simulink model "supercaps_dcbus_control"  (Simulink 7.2)
settings: Solver=ode45  StartTime=0.0  StopTime=1  RelTol=1e-3
undefined symbols (not defined in the file): C_dc, C_sto, L, V_dc0, V_sto0
libraries: simulink x1
settings Model: Creator=Pierre  LastModifiedBy=Pierre

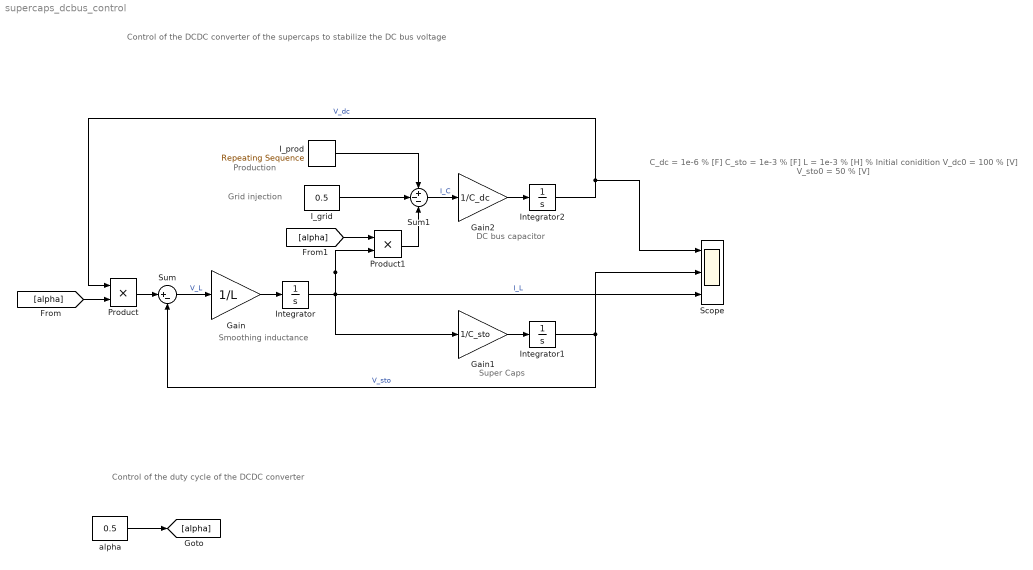
== system supercaps_dcbus_control ==
  note: Control of the DCDC converter of the supercaps
      | to stabilize the DC bus voltage
  note: Production
  note: C_dc = 1e-6 % [F]
      | C_sto = 1e-3 % [F]
      | L = 1e-3 % [H]
      |
      | % Initial conidition
      | V_dc0 = 100 % [V]
      | V_sto0 = 50 % [V]
  note: Grid injection
  note: Control of the duty cycle of the DCDC converter
  note: DC bus capacitor
  note: Super Caps
  note: Smoothing inductance
  Gain : Gain  Gain=1/L  ParameterDataType=sfix(16)  ParameterScaling=2^0  OutDataType=sfix(16)  OutScaling=2^0
  Gain1 : Gain  Gain=1/C_sto  ParameterDataType=sfix(16)  ParameterScaling=2^0  OutDataType=sfix(16)  OutScaling=2^0
  Gain2 : Gain  Gain=1/C_dc  ParameterDataType=sfix(16)  ParameterScaling=2^0  OutDataType=sfix(16)  OutScaling=2^0
  I_grid : Constant  Value=0.5  OutDataType=sfix(16)  OutScaling=2^0
  I_prod : simulink/Sources/Repeating Sequence  SystemSampleTime=-1  rep_seq_t=[0 .2 .4]  rep_seq_y=[0 2 0]
  Integrator : Integrator
  Integrator1 : Integrator  InitialCondition=V_sto0
  Integrator2 : Integrator  InitialCondition=V_dc0
  Product : Product  OutDataType=sfix(16)  OutScaling=2^0  RndMeth=Zero
  Product1 : Product  OutDataType=sfix(16)  OutScaling=2^0  RndMeth=Zero
  Scope : Scope  NumInputPorts=3
      settings: YMin=-5~-5~-5  YMax=5~5~5
  Sum : Sum  Inputs=|+-  OutDataType=sfix(16)  OutScaling=2^0
  Sum1 : Sum  Inputs=+--  OutDataType=sfix(16)  OutScaling=2^0
  alpha : Constant  Value=0.5  OutDataType=sfix(16)  OutScaling=2^0
  wires:
  Gain/1 -> Integrator/1
  Gain1/1 -> Integrator1/1
  Gain2/1 -> Integrator2/1
  Integrator1/1 -> Sum/2, Scope/2  "V_sto"
  Sum/1 -> Gain/1  "V_L"
  Product/1 -> Sum/1
  Integrator2/1 -> Product/1, Scope/1  "V_dc"
  I_prod/1 -> Sum1/1
  I_grid/1 -> Sum1/2
  alpha/1 -> [alpha]
  [alpha] -> Product/2
  [alpha] -> Product1/1
  Product1/1 -> Sum1/3
  Sum1/1 -> Gain2/1  "I_C"
  Integrator/1 -> Gain1/1, Product1/2, Scope/3  "I_L"
